simulink model "Automatisierung_subsystem_test"  (R2016b)
settings: Solver=VariableStepAuto  StartTime=0.0  StopTime=100.0  RelTol=1e-3
model workspace (MAT data in the model file):
  a = Simulink.Parameter
  a.DataType = 'auto'
  a.Dimensions = [0 0]
  b = Simulink.Parameter
  b.DataType = 'auto'
  b.Dimensions = [0 0]
settings Model: Creator=Fritz  LastModifiedBy=Fritz

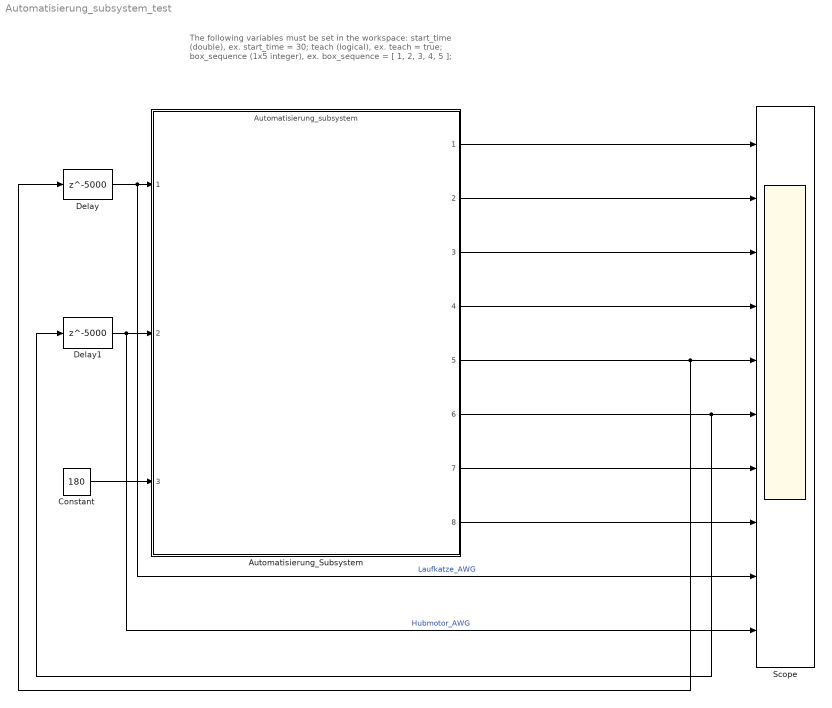
== system Automatisierung_subsystem_test ==
  note: The following variables must be set in the workspace:
      | start_time (double), ex. start_time = 30;
      | teach (logical), ex. teach = true;
      | box_sequence (1x5 integer), ex. box_sequence = [ 1, 2, 3, 4, 5 ];
  Automatisierung_Subsystem : ModelReference  ModelNameDialog=Automatisierung_subsystem.slx  SimulationMode=Normal  ModelReferenceVersion=1.74
  Constant : Constant  Value=180
  Delay : Delay  DelayLength=5000
  Delay1 : Delay  DelayLength=5000
  Scope : Scope  NumInputPorts=10
  wires:
  Automatisierung_Subsystem/1 -> Scope/1
  Automatisierung_Subsystem/2 -> Scope/2
  Automatisierung_Subsystem/3 -> Scope/3
  Automatisierung_Subsystem/4 -> Scope/4
  Automatisierung_Subsystem/5 -> Delay/1, Scope/5
  Automatisierung_Subsystem/7 -> Scope/7
  Automatisierung_Subsystem/8 -> Scope/8
  Delay/1 -> Scope/9, Automatisierung_Subsystem/1  "Laufkatze_AWG"
  Delay1/1 -> Scope/10, Automatisierung_Subsystem/2  "Hubmotor_AWG"
  Constant/1 -> Automatisierung_Subsystem/3
  Automatisierung_Subsystem/6 -> Delay1/1, Scope/6
